simulink subsystem "feed_forward_controller"  (R2025b)
settings: Solver=VariableStepAuto  StartTime=0.0  StopTime=10.0  RelTol=1e-3
undefined symbols (not defined in the file or in its folder): const_voltage, defined_maneuvers, dt_control, dt_data, max_thruster_force
settings Model: Creator=koryh  LastModifiedBy=koryh

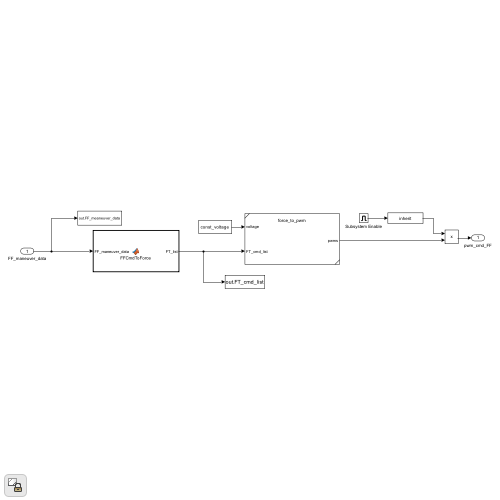
[thumbnail: Simulink's stored preview of the top-level diagram]
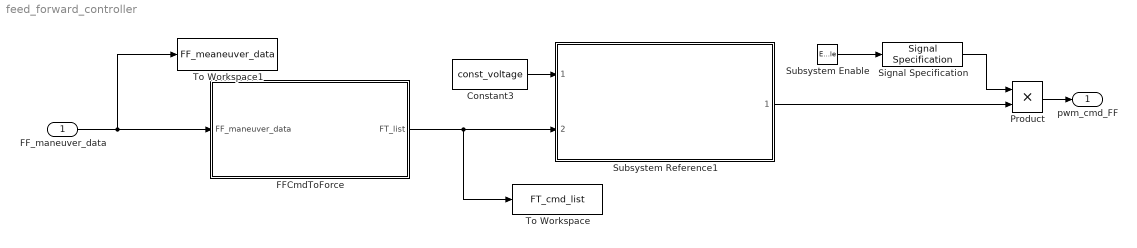
== system feed_forward_controller ==
  FF_maneuver_data : Inport  SampleTime=dt_control
  Subsystem Enable : EnablePort  PropagateVarSize=During execution  ShowOutputPort=on
  Constant3 : Constant  Value=const_voltage
  FFCmdToForce : MATLAB Function  TreatAsAtomicUnit=on
  Product : Product
  Signal Specification : SignalSpecification
  Subsystem Reference1 : Subsystem  ReferencedSubsystem=force_to_pwm
  To Workspace : ToWorkspace  VariableName=FT_cmd_list  SaveFormat=Timeseries  SampleTime=dt_data
  To Workspace1 : ToWorkspace  VariableName=FF_meaneuver_data  SaveFormat=Timeseries  SampleTime=dt_data
  pwm_cmd_FF : Outport  SampleTime=dt_control
  wires:
  FFCmdToForce/1(FT_list) -> To Workspace/1, Subsystem Reference1/2
  Constant3/1 -> Subsystem Reference1/1
  FF_maneuver_data/1 -> FFCmdToForce/1(FF_maneuver_data), To Workspace1/1
  Subsystem Reference1/1 -> Product/2
  Subsystem Enable/1 -> Signal Specification/1
  Signal Specification/1 -> Product/1
  Product/1 -> pwm_cmd_FF/1

== matlab function feed_forward_controller/FFCmdToForce ==
  data: FF_maneuver_data input; FT_list output size=[8,1]; max_thruster_force parameter; defined_maneuvers parameter
function FT_list = FFCmdToForce(FF_maneuver_data, max_thruster_force, defined_maneuvers)


FT_list = FFCmdToForce2(FF_maneuver_data,max_thruster_force, defined_maneuvers);
